simulink model "ACStesbed"  (R2015b)
settings: Solver=ode45  StartTime=0.0  StopTime=1500  FixedStep=0.02  RelTol=1e-3
StartFcn:
  | InitializeModel
values from neighbouring files (symbols this model uses):
  D = L+eye(3)    [controllability.m]    (also in func.m = skewsym(X(2:4))+eye(3); func1.m = skewsym(X(2:4))+eye(3); kab2.m = Dt'; sys1.m = skewsym(X0(2:4))+eye(3))
undefined symbols (not defined in the file or in its folder): DiscIntNeverNeededParam, e0_0, e1_0, e2_0, e3_0, OrbData, params
libraries: aerolibutil x16, vrlib x13, satellite_control_lib x8, dspmtrx3 x4, aerolibtransform2 x3, aerolib6dofsys x2, simulink x2, aerolib6dof2 x1, dspinverses x1, dspmathops x1
(part 1 of 2)
settings Model: Creator=DNikolaev  LastModifiedBy=DNikolaev
settings DataIOCC: SaveFormat=Array
settings DebuggingCC: UnderspecifiedInitializationDetection=Classic  MergeDetectMultiDrivingBlocksExec=none  SolverPrmCheckMsg=warning
settings HardwareCC: ProdBitPerPointer=32  ProdLargestAtomicFloat=None  ProdIntDivRoundTo=Undefined  ProdEndianess=Unspecified  ProdWordSize=32  ProdHWDeviceType=32-bit Generic
settings GRTTargetCC: GeneratePreprocessorConditionals=Disable all
settings ConfigComp: CovModelRefEnable=Off

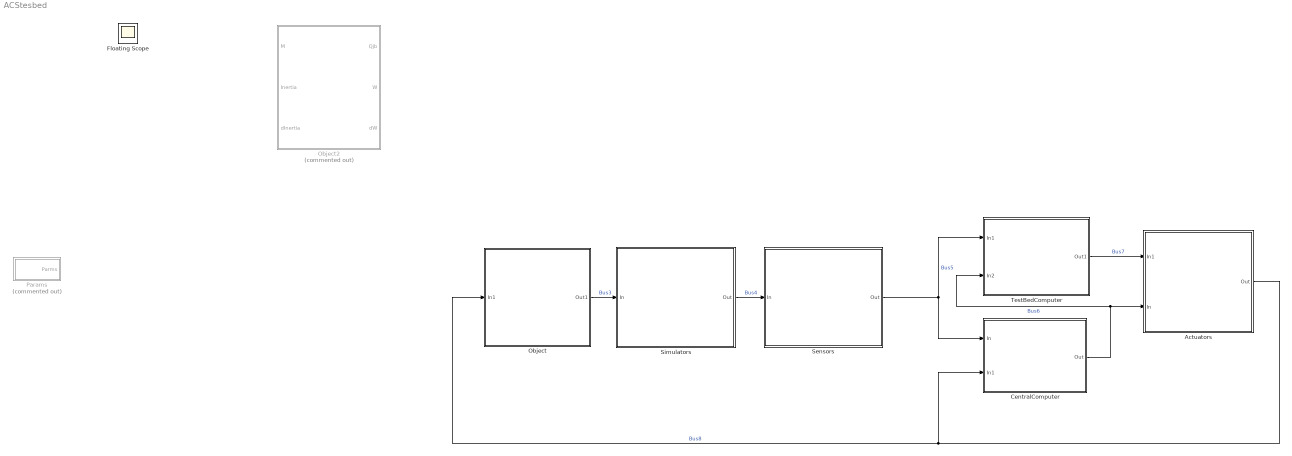
== system ACStesbed ==
  Actuators : Subsystem
      mask Display: image('ReactionWheel.gif','center','off')
  CentralComputer : Subsystem
      mask Display: image('cc.jpg')
  Object : Subsystem
      mask Display: image('abtestbed.jpg')
  Object2 : Subsystem  Commented=on
      mask Display: image('abtestbed.jpg')
  Params : Subsystem  Commented=on
  Sensors : Subsystem
      mask Display: image('gyro.jpg')
  Simulators : Subsystem
      mask Display: image('space.jpg')
  TestBedComputer : Subsystem  TreatAsAtomicUnit=on  SystemSampleTime=0.1
      mask Display: image('computer.jpg')
  Floating Scope : Scope
  wires:
  Simulators/1(Out) -> Sensors/1(In)  "Bus4"
  Sensors/1(Out) -> CentralComputer/1(In), TestBedComputer/1(In1)  "Bus5"
  Actuators/1(Out) -> Object/1(In1), CentralComputer/2(In1)  "Bus8"
  CentralComputer/1(Out) -> TestBedComputer/2(In2), Actuators/2(In)  "Bus6"
  TestBedComputer/1(Out1) -> Actuators/1(In1)  "Bus7"
  Object/1(Out1) -> Simulators/1(In)  "Bus3"

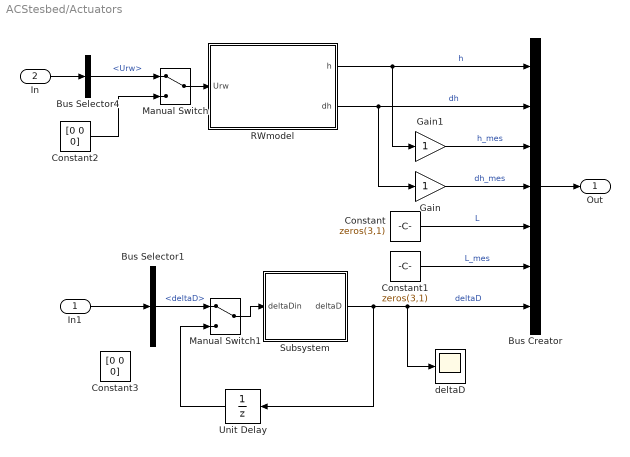
== system ACStesbed/Actuators ==
  In1 : Inport
  In : Inport  Port=2
  Bus Creator : BusCreator  Inputs=7
  Bus Selector1 : BusSelector  OutputSignals=deltaD
  Bus Selector4 : BusSelector  OutputSignals=Urw
  Constant : Constant  Value=zeros(3,1)
  Constant1 : Constant  Value=zeros(3,1)
  Constant2 : Constant  Value=[0 0 0]
  Constant3 : Constant  Value=[0 0 0]
  Gain : Gain
  Gain1 : Gain
  Manual Switch : ManualSwitch
  Manual Switch1 : ManualSwitch
  RWmodel : Subsystem
  Subsystem : Subsystem
  Unit Delay : UnitDelay  InitialCondition=[0 0 0]  SampleTime=-1
  deltaD : Scope
  Out : Outport
  wires:
  In/1 -> Bus Selector4/1
  Bus Creator/1 -> Out/1
  RWmodel/2(dh) -> Gain/1, Bus Creator/2  "dh"
  Constant/1 -> Bus Creator/5  "L"
  Constant1/1 -> Bus Creator/6  "L_mes"
  Subsystem/1(deltaD) -> Unit Delay/1, Bus Creator/7, deltaD/1  "deltaD"
  Bus Selector4/1 -> Manual Switch/1  "<Urw>"
  RWmodel/1(h) -> Bus Creator/1, Gain1/1  "h"
  Gain/1 -> Bus Creator/4  "dh_mes"
  Gain1/1 -> Bus Creator/3  "h_mes"
  In1/1 -> Bus Selector1/1
  Bus Selector1/1 -> Manual Switch1/1  "<deltaD>"
  Manual Switch/1 -> RWmodel/1(Urw)
  Constant2/1 -> Manual Switch/2
  Manual Switch1/1 -> Subsystem/1(deltaDin)
  Unit Delay/1 -> Manual Switch1/2

== system ACStesbed/CentralComputer ==
  In : Inport
  In1 : Inport  Port=2
  Bus Creator : BusCreator  Inputs=7
  Bus Selector : BusSelector  OutputSignals=W_mes,rj2000_mes,vj2000_mes,Qjb_starmes,B_mes,Sun_mag_angle_mes
  Bus Selector1 : BusSelector  OutputSignals=deltaD,h_mes,dh_mes
  ModelOfObject : Subsystem
  SPAttitude : Subsystem  Commented=on
  SatAttitude : Subsystem
  Out : Outport
  wires:
  In/1 -> Bus Selector/1
  Bus Creator/1 -> Out/1
  Bus Selector/1 -> SatAttitude/1(W_mes)  "<W_mes>"
  Bus Selector/2 -> SatAttitude/2(rj2000_mes)  "<rj2000_mes>"
  Bus Selector/3 -> SatAttitude/3(vj2000_mes)  "<vj2000_mes>"
  Bus Selector/4 -> SatAttitude/4(Qjb_starmes)  "<Qjb_starmes>"
  Bus Selector/5 -> SatAttitude/5(B_mes)  "<B_mes>"
  Bus Selector/6 -> SatAttitude/6(Rsun_mes)  "<Sun_mag_angle_mes>"
  ModelOfObject/1(J_est) -> Bus Creator/1, SatAttitude/7(J_mes)  "J_mes"
  SatAttitude/1(Urw) -> Bus Creator/2  "Urw"
  ModelOfObject/2(dJ_est) -> SatAttitude/8(dJ_mes)
  Bus Selector1/2 -> Bus Creator/7, SatAttitude/9(h_mes)  "<h_mes>"
  In1/1 -> Bus Selector1/1
  SatAttitude/3(Qjb_mes) -> Bus Creator/4  "Qjb_mes"
  SatAttitude/2(dW) -> Bus Creator/3  "dW"
  SatAttitude/4(Qob_mes) -> Bus Creator/5  "Qob_mes"
  Bus Selector1/1 -> ModelOfObject/1(deltaD)  "<deltaD>"
  Bus Selector1/3 -> Bus Creator/6  "<dh_mes>"

== system ACStesbed/Object ==
  In1 : Inport
  Bus Creator{,1..3} (4 alike) : BusCreator  Inputs=2
  Bus Selector : BusSelector  OutputSignals=Bus8.deltaD
  Bus Selector1 : BusSelector  OutputSignals=vj2000,j2000
  From Workspace : FromWorkspace  VariableName=InData  OutDataTypeStr=Bus: BusObject  SampleTime=0  OutputAfterFinalValue=Holding final value
  Inertia : Subsystem
  OrbitalBasis : Subsystem
  TestBedDynamics : Subsystem
      mask Display: image('abtestbed.jpg')
  Torques : Subsystem
  Out1 : Outport
  wires:
  TestBedDynamics/1(Qjb) -> Bus Creator/1  "Qjb"
  TestBedDynamics/2(Omega) -> Bus Creator/2  "W"
  Inertia/1(Inertia) -> TestBedDynamics/2(Inertia)
  Torques/1(T) -> TestBedDynamics/1(M)
  From Workspace/1 -> Bus Selector1/1, Bus Creator1/2  "Bus1"
  Bus Selector1/1 -> OrbitalBasis/1(vj2000)  "<vj2000>"
  Bus Selector1/2 -> OrbitalBasis/2(rj2000)  "<j2000>"
  Bus Creator/1 -> Bus Creator2/1, Bus Creator1/1
  Bus Creator1/1 -> Out1/1  "Bus3"
  Bus Creator2/1 -> Torques/1(InData)
  Inertia/2(dInertia) -> TestBedDynamics/3(dInertia)
  In1/1 -> Bus Creator3/1
  OrbitalBasis/1(Qjo) -> Bus Creator3/2
  Bus Creator3/1 -> Bus Selector/1, Bus Creator2/2
  Bus Selector/1 -> Inertia/1(deltaD)  "<deltaD>"

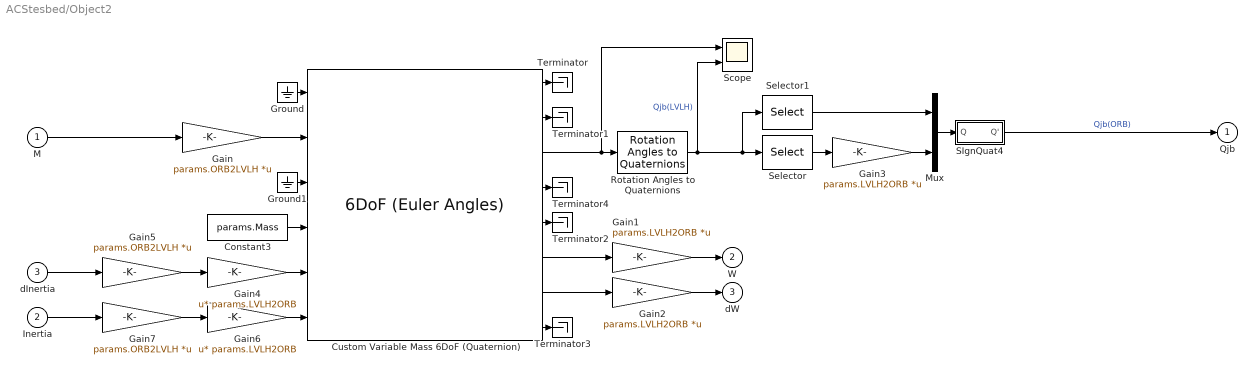
== system ACStesbed/Object2 ==
  M : Inport
  Inertia : Inport  Port=2
  dInertia : Inport  Port=3
  Constant3 : Constant  Value=params.Mass
  Custom Variable Mass 6DoF (Quaternion) : aerolib6dof2/6DoF (Euler Angles)  units=Metric (MKS)  mtype=Custom Variable  rep=Quaternion  xme_0=[0 0 0]  Vm_0=[0 0 0]  eul_0=[params.roll,params.pitch,params.yaw]  pm_0=params.ORB2LVLH*params.W_b  mass_0=1.0  mass_e=0  mass_f=0  inertia=eye(3)  inertia_e=eye(3)  inertia_f=eye(3)  k_quat=1.0
  Gain : Gain  Gain=params.ORB2LVLH  Multiplication=Matrix(K*u) (u vector)
  Gain1 : Gain  Gain=params.LVLH2ORB  Multiplication=Matrix(K*u) (u vector)
  Gain2 : Gain  Gain=params.LVLH2ORB  Multiplication=Matrix(K*u) (u vector)
  Gain3 : Gain  Gain=params.LVLH2ORB  Multiplication=Matrix(K*u) (u vector)
  Gain4 : Gain  Gain=params.LVLH2ORB  Multiplication=Matrix(u*K)
  Gain5 : Gain  Gain=params.ORB2LVLH  Multiplication=Matrix(K*u)
  Gain6 : Gain  Gain=params.LVLH2ORB  Multiplication=Matrix(u*K)
  Gain7 : Gain  Gain=params.ORB2LVLH  Multiplication=Matrix(K*u)
  Ground : Ground
  Ground1 : Ground
  Mux : Mux  Inputs=2
  Rotation Angles to Quaternions : aerolibtransform2/Rotation Angles to Quaternions  rotationOrder=XYZ
  SIgnQuat4 : Subsystem
  Scope : Scope  NumInputPorts=2
  Selector : Selector  InputPortWidth=4  IndexOptions=Index vector (dialog)  Indices=[2 3 4]  OutputSizes=1
  Selector1 : Selector  InputPortWidth=4  IndexOptions=Index vector (dialog)  Indices=1  OutputSizes=1
  Terminator{,1..4} (5 alike) : Terminator
  Qjb : Outport
  W : Outport  Port=2
  dW : Outport  Port=3
  wires:
  SIgnQuat4/1(Q') -> Qjb/1  "Qjb(ORB)"
  Mux/1 -> SIgnQuat4/1(Q)
  Constant3/1 -> Custom Variable Mass 6DoF (Quaternion)/4
  Gain6/1 -> Custom Variable Mass 6DoF (Quaternion)/6
  Gain7/1 -> Gain6/1
  Gain4/1 -> Custom Variable Mass 6DoF (Quaternion)/5
  Gain5/1 -> Gain4/1
  Gain3/1 -> Mux/2
  Selector1/1 -> Mux/1
  Selector/1 -> Gain3/1
  Inertia/1 -> Gain7/1
  Custom Variable Mass 6DoF (Quaternion)/3 -> Rotation Angles to Quaternions/1, Scope/1
  Gain2/1 -> dW/1
  Gain1/1 -> W/1
  Gain/1 -> Custom Variable Mass 6DoF (Quaternion)/2
  Custom Variable Mass 6DoF (Quaternion)/4 -> Terminator4/1
  dInertia/1 -> Gain5/1
  M/1 -> Gain/1
  Rotation Angles to Quaternions/1 -> Selector/1, Selector1/1, Scope/2  "Qjb(LVLH)"
  Custom Variable Mass 6DoF (Quaternion)/8 -> Terminator3/1
  Ground/1 -> Custom Variable Mass 6DoF (Quaternion)/1
  Custom Variable Mass 6DoF (Quaternion)/5 -> Terminator2/1
  Custom Variable Mass 6DoF (Quaternion)/1 -> Terminator/1
  Custom Variable Mass 6DoF (Quaternion)/7 -> Gain2/1
  Custom Variable Mass 6DoF (Quaternion)/6 -> Gain1/1
  Ground1/1 -> Custom Variable Mass 6DoF (Quaternion)/3
  Custom Variable Mass 6DoF (Quaternion)/2 -> Terminator1/1

== system ACStesbed/Params ==
  Bus Creator : BusCreator  Inputs=6
  Constant : Constant  Value=params.invJ_b
  Constant1 : Constant  Value=params.J_b
  Constant2 : Constant  Value=params.Nob
  Constant3 : Constant  Value=params.Mass
  Constant5 : Constant  Value=params.W_b
  Parms : Outport
  wires:
  Bus Creator/1 -> Parms/1
  Constant5/1 -> Bus Creator/5  "W_b_0"
  Constant2/1 -> Bus Creator/4  "Nob_0"
  Constant1/1 -> Bus Creator/2  "Inertia_0"
  Constant/1 -> Bus Creator/1  "invInertia_0"
  Constant3/1 -> Bus Creator/3  "Mass"

== system ACStesbed/Sensors ==
  In : Inport
  Bus Creator : BusCreator  Inputs=6
  Bus Selector4 : BusSelector  OutputSignals=j2000,vj2000,W,B,Qjb,Rsun
  MagnSensor : Subsystem
  PositionSensor : Subsystem
  RateSensor : Subsystem
      mask Display: text(0.5,0.5,'\omega=(I_3+S)\omega^{true}+\beta^{true}+\eta_\nu','hor','center','texmode','on')
  SIgnQuat : Subsystem
  StarSensor : Subsystem
  SunSensor : Subsystem
  Out : Outport
  wires:
  Bus Creator/1 -> Out/1
  In/1 -> Bus Selector4/1
  Bus Selector4/3 -> RateSensor/1(W)  "<W>"
  Bus Selector4/4 -> MagnSensor/1(Bms)  "<B>"
  Bus Selector4/1 -> SunSensor/2(rj2000), PositionSensor/1(rj2000)  "<j2000>"
  Bus Selector4/2 -> PositionSensor/2(vj2000)  "<vj2000>"
  Bus Selector4/5 -> SunSensor/1(Qjb), StarSensor/1(Qjb)  "<Qjb>"
  StarSensor/1(Qjb_mes) -> SIgnQuat/1(Q)
  MagnSensor/1(B_mes) -> Bus Creator/4  "B_mes"
  RateSensor/1(W_mes) -> Bus Creator/3  "W_mes"
  PositionSensor/2(vj2000_mes) -> Bus Creator/2  "vj2000_mes"
  PositionSensor/1(rj2000_mes) -> Bus Creator/1  "rj2000_mes"
  SIgnQuat/1(Q') -> Bus Creator/5  "Qjb_starmes"
  Bus Selector4/6 -> SunSensor/3(Rsun)  "<Rsun>"
  SunSensor/1(Sun_mag_angle_mes) -> Bus Creator/6

== system ACStesbed/Simulators ==
  In : Inport
  Bus Creator : BusCreator  Inputs=7
  Bus Selector1 : BusSelector  OutputSignals=signal1.W,signal1.Qjb
  Bus Selector4 : BusSelector  OutputSignals=Bus1.vj2000,Bus1.j2000,Bus1.rsun
  MagnSim : Subsystem
  StarSim : Subsystem
  SunSim : Subsystem
  Out : Outport
  wires:
  Bus Selector4/1 -> Bus Creator/1  "<vj2000>"
  In/1 -> Bus Selector1/1, Bus Selector4/1
  Bus Selector4/2 -> MagnSim/1(j2000), Bus Creator/2  "<j2000>"
  StarSim/1(Out) -> Bus Creator/3  "Stars"
  MagnSim/1(B) -> Bus Creator/4  "B"
  SunSim/1(Rsun_out) -> Bus Creator/5  "Rsun"
  Bus Creator/1 -> Out/1
  Bus Selector4/3 -> SunSim/1(Rsun)  "<rsun>"
  Bus Selector1/1 -> Bus Creator/6  "<W>"
  Bus Selector1/2 -> StarSim/1(In), Bus Creator/7  "<Qjb>"

== system ACStesbed/TestBedComputer ==
  In1 : Inport
  In2 : Inport  Port=2
  Bus Creator2 : BusCreator  Inputs=1
  Bus Selector3 : BusSelector  OutputSignals=rj2000_mes,vj2000_mes,W_mes
  Bus Selector4 : BusSelector  OutputSignals=Qob_mes,J_mes,dW,Urw,dh_mes,h_mes
  Constant8 : Constant  Value=params.g
  HorEst : Subsystem
  Mux : Mux  Inputs=2
  Quaternion Rotation2 : aerolibutil/Quaternion Rotation
  VerEst : Subsystem
  Out1 : Outport
  wires:
  In1/1 -> Bus Selector3/1
  In2/1 -> Bus Selector4/1
  Bus Creator2/1 -> Out1/1
  Mux/1 -> Bus Creator2/1  "deltaD"
  Bus Selector4/1 -> Quaternion Rotation2/1  "<Qob_mes>"
  Bus Selector4/3 -> HorEst/2(dW)  "<dW>"
  HorEst/1(deltaD12) -> Mux/1
  Constant8/1 -> Quaternion Rotation2/2  "g"
  Quaternion Rotation2/1 -> VerEst/1(gb), HorEst/1(gb)
  Bus Selector4/4 -> ?  "<Urw>"
  Bus Selector4/2 -> VerEst/2(J)  "<J_mes>"
  Bus Selector4/5 -> VerEst/3(dh)  "<dh_mes>"
  Bus Selector4/6 -> VerEst/4(h)  "<h_mes>"
  Bus Selector3/3 -> VerEst/5(W)  "<W_mes>"
  VerEst/1(Rz_est) -> ?  "Rz_est"

== system ACStesbed/Actuators/RWmodel ==
  Urw : Inport
  Gain1 : Gain
  Integrator Limited : Integrator  InitialCondition=[0 0 0]  LimitOutput=on  UpperSaturationLimit=100  LowerSaturationLimit=-100
  Rate Transition : RateTransition  OutPortSampleTime=0.01
  Saturation : Saturate
  "dh, h" : Scope  NumInputPorts=2
  h : Outport
  dh : Outport  Port=2
  wires:
  Urw/1 -> Rate Transition/1
  Integrator Limited/1 -> "dh, h"/2, h/1  "h"
  Gain1/1 -> Saturation/1  "dh"
  Saturation/1 -> dh/1
  Rate Transition/1 -> "dh, h"/1, Gain1/1, Integrator Limited/1  "dh"

== system ACStesbed/Actuators/Subsystem ==
  deltaDin : Inport
  Rate Transition : RateTransition  OutPortSampleTime=0.01
  deltaD : Outport
  wires:
  Rate Transition/1 -> deltaD/1  "deltaD"
  deltaDin/1 -> Rate Transition/1

== system ACStesbed/CentralComputer/ModelOfObject ==
  deltaD : Inport
  ChangeMe1 : Constant  Value=zeros(3,3)
  ChangeMe4 : Constant  Value=zeros(3,3)
  Inertia : Subsystem
  J_est : Outport
  dJ_est : Outport  Port=2
  R_est : Outport  Port=3
  wires:
  deltaD/1 -> Inertia/1(deltaD)
  ChangeMe1/1 -> dJ_est/1
  Inertia/1(Inertia) -> J_est/1
  ChangeMe4/1 -> R_est/1

== system ACStesbed/CentralComputer/SPAttitude ==
  In1 : Inport
  Out1 : Outport
  wires:
  In1/1 -> Out1/1

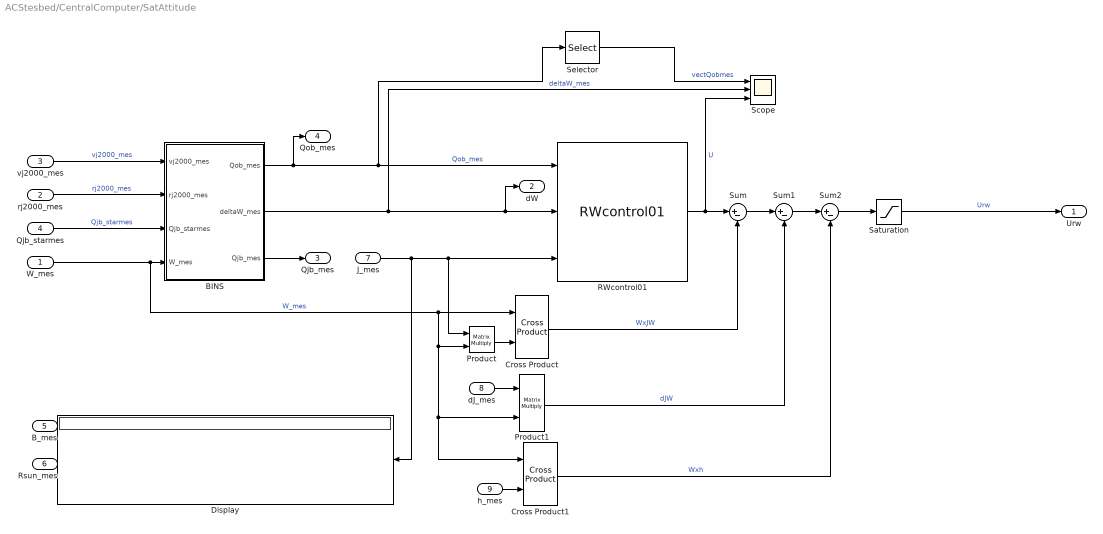
== system ACStesbed/CentralComputer/SatAttitude ==
  W_mes : Inport
  rj2000_mes : Inport  Port=2
  vj2000_mes : Inport  Port=3
  Qjb_starmes : Inport  Port=4
  B_mes : Inport  Port=5
  Rsun_mes : Inport  Port=6
  J_mes : Inport  Port=7
  dJ_mes : Inport  Port=8
  h_mes : Inport  Port=9
  BINS : Subsystem
  Cross Product : vrlib/Utilities/Cross Product
  Cross Product1 : vrlib/Utilities/Cross Product
  Display : Display
  Product : Product  Multiplication=Matrix(*)
  Product1 : Product  Multiplication=Matrix(*)
  RWcontrol01 : satellite_control_lib/RWcontrol01  Kq=params.K1acs  Kw=params.K2acs
  Saturation : Saturate
  Scope : Scope  NumInputPorts=3
  Selector : Selector  InputPortWidth=4  IndexOptions=Index vector (dialog)  Indices=[2 3 4]  OutputSizes=1
  Sum : Sum  Inputs=|+-
  Sum1 : Sum  Inputs=|+-
  Sum2 : Sum  Inputs=|+-
  Urw : Outport
  dW : Outport  Port=2
  Qjb_mes : Outport  Port=3
  Qob_mes : Outport  Port=4
  wires:
  RWcontrol01/1 -> Scope/3, Sum/1  "U"
  vj2000_mes/1 -> BINS/1(vj2000_mes)  "vj2000_mes"
  rj2000_mes/1 -> BINS/2(rj2000_mes)  "rj2000_mes"
  Qjb_starmes/1 -> BINS/3(Qjb_starmes)  "Qjb_starmes"
  W_mes/1 -> Product/2, Product1/2, Cross Product1/1, Cross Product/1, BINS/4(W_mes)  "W_mes"
  J_mes/1 -> Display/1, Product/1, RWcontrol01/3
  BINS/1(Qob_mes) -> Qob_mes/1, Selector/1, RWcontrol01/1  "Qob_mes"
  BINS/2(deltaW_mes) -> Scope/2, dW/1, RWcontrol01/2  "deltaW_mes"
  Product/1 -> Cross Product/2
  Cross Product/1 -> Sum/2  "WxJW"
  Product1/1 -> Sum1/2  "dJW"
  Cross Product1/1 -> Sum2/2  "Wxh"
  Sum/1 -> Sum1/1
  Sum1/1 -> Sum2/1
  Sum2/1 -> Saturation/1
  h_mes/1 -> Cross Product1/2
  dJ_mes/1 -> Product1/1
  BINS/3(Qjb_mes) -> Qjb_mes/1
  Saturation/1 -> Urw/1  "Urw"
  Selector/1 -> Scope/1  "vectQobmes"

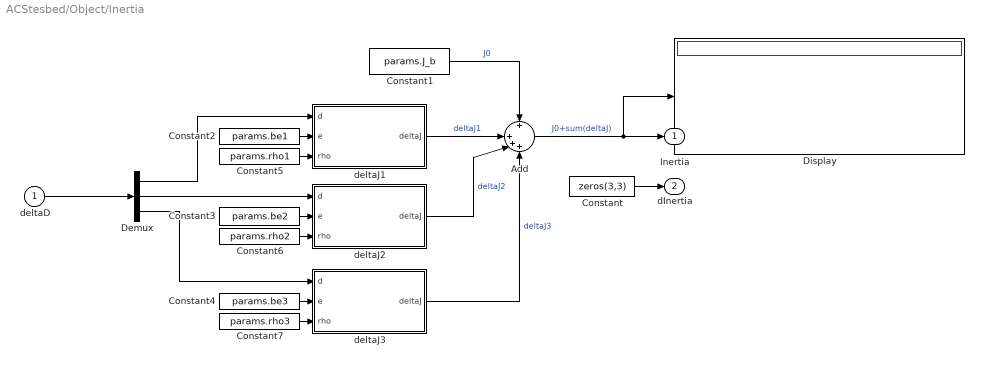
== system ACStesbed/Object/Inertia ==
  deltaD : Inport
  Add : Sum  Inputs=+|+++
  Constant : Constant  Value=zeros(3,3)
  Constant1 : Constant  Value=params.J_b
  Constant2 : Constant  Value=params.be1
  Constant3 : Constant  Value=params.be2
  Constant4 : Constant  Value=params.be3
  Constant5 : Constant  Value=params.rho1
  Constant6 : Constant  Value=params.rho2
  Constant7 : Constant  Value=params.rho3
  Demux : Demux  Outputs=3
  Display : Display
  deltaJ1 : Subsystem
  deltaJ2 : Subsystem
  deltaJ3 : Subsystem
  Inertia : Outport
  dInertia : Outport  Port=2
  wires:
  Constant/1 -> dInertia/1
  Constant1/1 -> Add/1  "J0"
  deltaD/1 -> Demux/1
  deltaJ1/1(deltaJ) -> Add/2  "deltaJ1"
  deltaJ2/1(deltaJ) -> Add/3  "deltaJ2"
  deltaJ3/1(deltaJ) -> Add/4  "deltaJ3"
  Add/1 -> Display/1, Inertia/1  "J0+sum(deltaJ)"
  Demux/1 -> deltaJ1/1(d)
  Demux/2 -> deltaJ2/1(d)
  Demux/3 -> deltaJ3/1(d)
  Constant4/1 -> deltaJ3/2(e)
  Constant3/1 -> deltaJ2/2(e)
  Constant2/1 -> deltaJ1/2(e)
  Constant7/1 -> deltaJ3/3(rho)
  Constant6/1 -> deltaJ2/3(rho)
  Constant5/1 -> deltaJ1/3(rho)

== system ACStesbed/Object/OrbitalBasis ==
  vj2000 : Inport
  rj2000 : Inport  Port=2
  Cross Product : vrlib/Utilities/Cross Product
  Cross Product1 : vrlib/Utilities/Cross Product
  Direction Cosine Matrix to Quaternions : aerolibtransform2/Direction Cosine Matrix  to Quaternions
  Matrix Concatenate : Concatenate  NumInputs=3  Mode=Multidimensional array  ConcatenateDimension=2
  Normalize Vector : vrlib/Utilities/Normalize Vector  maxzero=0.00001
  Normalize Vector1 : vrlib/Utilities/Normalize Vector  maxzero=0.00001
  Quaternion Conjugate : aerolibutil/Quaternion Conjugate
  Qjo : Outport
  wires:
  Cross Product1/1 -> Matrix Concatenate/1  "iorb"
  Normalize Vector/1 -> Matrix Concatenate/2, Cross Product1/1  "jorb"
  Matrix Concatenate/1 -> Direction Cosine Matrix to Quaternions/1  "DCMjo"
  rj2000/1 -> Normalize Vector/1, Cross Product/2
  vj2000/1 -> Cross Product/1
  Direction Cosine Matrix to Quaternions/1 -> Quaternion Conjugate/1  "Qjo(in J frame)"
  Normalize Vector1/1 -> Matrix Concatenate/3, Cross Product1/2  "korb"
  Cross Product/1 -> Normalize Vector1/1
  Quaternion Conjugate/1 -> Qjo/1  "Qjo"

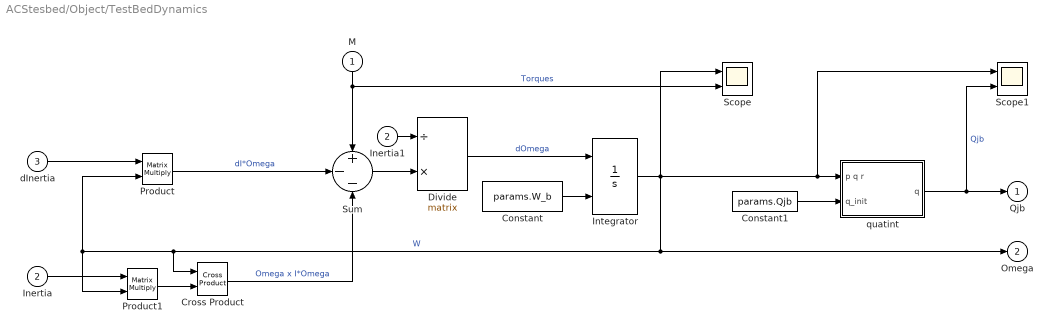
== system ACStesbed/Object/TestBedDynamics ==
  M : Inport
  Inertia : Inport  Port=2
  dInertia : Inport  Port=3
  Constant : Constant  Value=params.W_b
  Constant1 : Constant  Value=params.Qjb
  Cross Product : vrlib/Utilities/Cross Product
  Divide : Product  Inputs=/*  Multiplication=Matrix(*)
  Inertia1 : InportShadow  Port=2
  Integrator : Integrator  InitialConditionSource=external
  Product : Product  Multiplication=Matrix(*)
  Product1 : Product  Multiplication=Matrix(*)
  Scope : Scope  NumInputPorts=2
  Scope1 : Scope  NumInputPorts=2
  Sum : Sum  Inputs=+--
  quatint : Subsystem
  Qjb : Outport
  Omega : Outport  Port=2
  wires:
  Sum/1 -> Divide/2
  Inertia1/1 -> Divide/1
  Divide/1 -> Integrator/1  "dOmega"
  Constant/1 -> Integrator/2
  Product/1 -> Sum/2  "dI*Omega"
  dInertia/1 -> Product/1
  Constant1/1 -> quatint/2(q_init)
  quatint/1(q) -> Scope1/2, Qjb/1  "Qjb"
  Inertia/1 -> Product1/1
  Product1/1 -> Cross Product/2
  Cross Product/1 -> Sum/3  "Omega x I*Omega"
  Integrator/1 -> Scope/1, Scope1/1, quatint/1(p q r), Cross Product/1, Product/2, Product1/2, Omega/1  "W"
  M/1 -> Scope/2, Sum/1  "Torques"

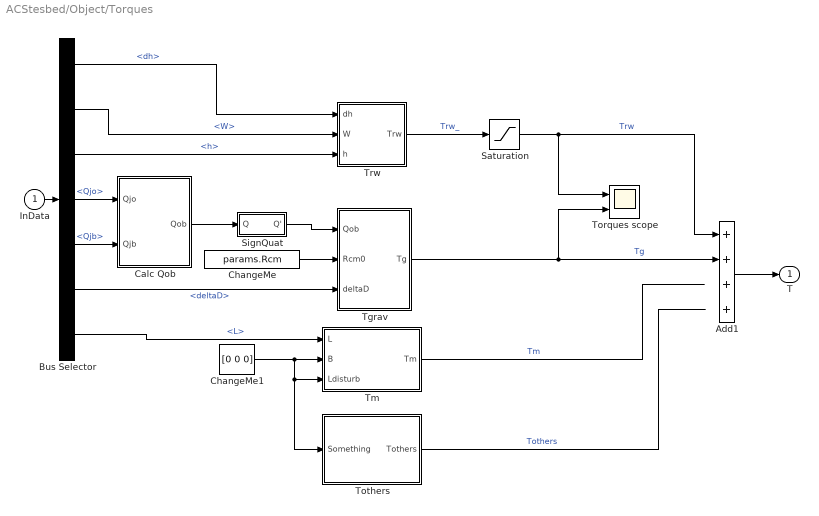
== system ACStesbed/Object/Torques ==
  InData : Inport
  Add1 : Sum  Inputs=4
  Bus Selector : BusSelector  OutputSignals=signal2.Bus8.dh,signal1.W,signal2.Bus8.h,signal2.Qjo,signal1.Qjb,signal2.Bus8.deltaD,signal2.Bus8.L
  Calc Qob : Subsystem
  ChangeMe : Constant  Value=params.Rcm
  ChangeMe1 : Constant  Value=[0 0 0]
  Saturation : Saturate  UpperLimit=1  LowerLimit=-1
  SignQuat : Subsystem
  Tgrav : Subsystem
  Tm : Subsystem
  Torques scope : Scope  NumInputPorts=2
  Tothers : Subsystem
  Trw : Subsystem
  T : Outport
  wires:
  InData/1 -> Bus Selector/1
  Bus Selector/7 -> Tm/1(L)  "<L>"
  Bus Selector/6 -> Tgrav/3(deltaD)  "<deltaD>"
  Add1/1 -> T/1
  Bus Selector/1 -> Trw/1(dh)  "<dh>"
  Bus Selector/2 -> Trw/2(W)  "<W>"
  Bus Selector/3 -> Trw/3(h)  "<h>"
  Trw/1(Trw) -> Saturation/1  "Trw_"
  Tgrav/1(Tg) -> Torques scope/2, Add1/2  "Tg"
  Tm/1(Tm) -> ?  "Tm"
  Tothers/1(Tothers) -> ?  "Tothers"
  ChangeMe1/1 -> Tothers/1(Something), Tm/3(Ldisturb), Tm/2(B)
  Saturation/1 -> Torques scope/1, Add1/1  "Trw"
  ChangeMe/1 -> Tgrav/2(Rcm0)
  Calc Qob/1(Qob) -> SignQuat/1(Q)
  Bus Selector/5 -> Calc Qob/2(Qjb)  "<Qjb>"
  Bus Selector/4 -> Calc Qob/1(Qjo)  "<Qjo>"
  SignQuat/1(Q') -> Tgrav/1(Qob)

== system ACStesbed/Object2/SIgnQuat4 ==
  Q : Inport
  Constant : Constant
  Constant1 : Constant  Value=-1
  Product : Product
  Selector2 : Selector  InputPortWidth=4  IndexOptions=Index vector (dialog)  Indices=[1]  OutputSizes=1
  Switch : Switch
  Q' : Outport
  wires:
  Constant1/1 -> Switch/3
  Constant/1 -> Switch/1
  Selector2/1 -> Switch/2
  Switch/1 -> Product/1
  Product/1 -> Q'/1
  Q/1 -> Selector2/1, Product/2

== system ACStesbed/Sensors/MagnSensor ==
  note: B_mes=A*B+b+w
  Bms : Inport
  A : Constant  Value=diag([1 1 1])
  Matrix Multiply : Product  Multiplication=Matrix(*)
  Random Noise : RandomNumber  Variance=params.MS_varianse  SampleTime=params.MS_sample_time
  Reshape : Reshape  OutputDimensionality=Column vector (2-D)
  Sum : Sum  Inputs=|++
  Sum1 : Sum  Inputs=|++
  Zero-Order Hold : ZeroOrderHold  SampleTime=params.SS_sample_time
  b : Constant  Value=[0;0;0]
  B_mes : Outport
  wires:
  Random Noise/1 -> Sum/2  "w"
  Bms/1 -> Zero-Order Hold/1
  Sum/1 -> B_mes/1  "B_mes"
  A/1 -> Matrix Multiply/1  "A"
  Matrix Multiply/1 -> Sum1/1
  Reshape/1 -> Matrix Multiply/2  "B"
  b/1 -> Sum1/2  "b"
  Zero-Order Hold/1 -> Reshape/1
  Sum1/1 -> Sum/1

== system ACStesbed/Sensors/PositionSensor ==
  rj2000 : Inport
  vj2000 : Inport  Port=2
  Noise : Constant  Value=[0 0 0]
  Noise1 : Constant  Value=[0 0 0]
  Sum : Sum  Inputs=|++
  Sum1 : Sum  Inputs=|++
  Zero-Order Hold : ZeroOrderHold  SampleTime=0.1
  Zero-Order Hold1 : ZeroOrderHold  SampleTime=0.1
  rj2000_mes : Outport
  vj2000_mes : Outport  Port=2
  wires:
  rj2000/1 -> Sum/1
  Noise/1 -> Sum/2
  Sum/1 -> Zero-Order Hold/1
  Zero-Order Hold/1 -> rj2000_mes/1
  vj2000/1 -> Sum1/1
  Noise1/1 -> Sum1/2
  Sum1/1 -> Zero-Order Hold1/1
  Zero-Order Hold1/1 -> vj2000_mes/1

== system ACStesbed/Sensors/RateSensor ==
  W : Inport
  Add : Sum
  Band-Limited White Noise : simulink/Sources/Band-Limited White Noise  Cov=params.VarRSB/0.1  Ts=0.1  seed=[23341]
  Band-Limited White Noise1 : simulink/Sources/Band-Limited White Noise  Cov=params.VarRSN/0.1  Ts=0.1  seed=[23341]
  Constant : Constant  Value=params.RSSE
  I3 : dspmtrx3/Constant Diagonal Matrix  q=ones(1,3)  frame=off  dataType=Inherit from 'Constant(s) along diagonal'  isSigned=on  wordLen=16  udDataType=sfix(16)  fracBitsMode=Best precision  numFracBits=15
  Integrator : Integrator
  Manual Switch : ManualSwitch
  Product : Product  Multiplication=Matrix(*)
  Sum : Sum  Inputs=|++
  Sum1 : Sum  Inputs=|++
  Zero-Order Hold : ZeroOrderHold  SampleTime=0.1
  Zero-Order Hold1 : ZeroOrderHold  SampleTime=0.1
  W_mes : Outport
  wires:
  W/1 -> Zero-Order Hold1/1, Product/2
  Sum/1 -> Zero-Order Hold/1
  Zero-Order Hold/1 -> Manual Switch/2
  Sum1/1 -> Sum/1
  I3/1 -> Add/1
  Constant/1 -> Add/2
  Add/1 -> Product/1
  Product/1 -> Sum1/1
  Band-Limited White Noise1/1 -> Sum/2  "noise"
  Integrator/1 -> Sum1/2  "Bias"
  Band-Limited White Noise/1 -> Integrator/1  "dBias"
  Manual Switch/1 -> W_mes/1
  Zero-Order Hold1/1 -> Manual Switch/1

== system ACStesbed/Sensors/SIgnQuat ==
  Q : Inport
  Product : Product
  Selector2 : Selector  InputPortWidth=4  IndexOptions=Index vector (dialog)  Indices=[1]  OutputSizes=1
  Sign : Signum
  Q' : Outport
  wires:
  Q/1 -> Product/2, Selector2/1
  Product/1 -> Q'/1
  Sign/1 -> Product/1
  Selector2/1 -> Sign/1

== system ACStesbed/Sensors/StarSensor ==
  Qjb : Inport
  Noise : Constant  Value=[1 0 0 0]
  Quaternion Multiplication : aerolibutil/Quaternion Multiplication
  Zero-Order Hold : ZeroOrderHold  SampleTime=0.1
  Qjb_mes : Outport
  wires:
  Zero-Order Hold/1 -> Qjb_mes/1
  Qjb/1 -> Quaternion Multiplication/1
  Noise/1 -> Quaternion Multiplication/2
  Quaternion Multiplication/1 -> Zero-Order Hold/1

== system ACStesbed/Sensors/SunSensor ==
  Qjb : Inport
  rj2000 : Inport  Port=2
  Rsun : Inport  Port=3
  Constant : Constant  Value=params.Qb_ss
  DigitalSunSensor : Subsystem
  Gain : Gain  Gain=params.au2km
  Quaternion Multiplication : aerolibutil/Quaternion Multiplication
  Quaternion Rotation : aerolibutil/Quaternion Rotation
  Subtract : Sum  Inputs=|+-
  Sun_mag_angle_mes : Outport
  wires:
  Quaternion Rotation/1 -> DigitalSunSensor/1(Rsun_ss)  "Rsun_ss"
  Gain/1 -> Subtract/1
  Subtract/1 -> Quaternion Rotation/2  "Rsun_j"
  Quaternion Multiplication/1 -> Quaternion Rotation/1  "Qj_ss"
  Rsun/1 -> Gain/1
  DigitalSunSensor/1(Sun_mag_angle_mes) -> Sun_mag_angle_mes/1  "Sun_mag_angle_mes"
  Constant/1 -> Quaternion Multiplication/2
  rj2000/1 -> Subtract/2
  Qjb/1 -> Quaternion Multiplication/1

== system ACStesbed/Simulators/MagnSim ==
  j2000 : Inport
  B : Outport
  wires:
  j2000/1 -> B/1

== system ACStesbed/Simulators/StarSim ==
  In : Inport
  Out : Outport
  wires:
  In/1 -> Out/1

== system ACStesbed/Simulators/SunSim ==
  Rsun : Inport
  Rsun_out : Outport
  wires:
  Rsun/1 -> Rsun_out/1

== system ACStesbed/TestBedComputer/HorEst ==
  gb : Inport
  dW : Inport  Port=2
  Constant13 : Constant  Value=params.invU
  Gain : Gain  Gain=-params.Mass
  Gain1 : Gain  Gain=params.Mass/params.bmass+3
  Product8 : Product  Inputs=3  Multiplication=Matrix(*)
  Pseudoinverse : dspinverses/Pseudoinverse  wanterr=off
  Selector : Selector  InputPortWidth=3  IndexOptions=Index vector (dialog)  Indices=[1 2]  OutputSizes=1
  Skew-symmetric matrix2 : satellite_control_lib/Skew-symmetric matrix
  Subsystem : Subsystem
  deltaD HorEst : Scope
  tau_b : Scope
  deltaD12 : Outport
  wires:
  gb/1 -> Skew-symmetric matrix2/1, Subsystem/2(gb)  "gb"
  Skew-symmetric matrix2/1 -> Gain/1  "G"
  Pseudoinverse/1 -> Product8/2  "psinvG"
  dW/1 -> Subsystem/3(dW)
  Subsystem/1(taub) -> Product8/3, tau_b/1
  Constant13/1 -> Product8/1
  Product8/1 -> Gain1/1
  Selector/1 -> deltaD12/1
  Gain/1 -> Subsystem/1(G), Pseudoinverse/1  "G"
  Gain1/1 -> deltaD HorEst/1, Selector/1

== system ACStesbed/TestBedComputer/VerEst ==
  gb : Inport
  J : Inport  Port=2
  dh : Inport  Port=3
  h : Inport  Port=4
  W : Inport  Port=5
  Constant1 : Constant  Value=params.Mass
  Display : Display
  Scope : Scope
  Scope1 : Scope
  Unit Delay : UnitDelay  InitialCondition=0.001  SampleTime=-1
  Unit Delay1 : UnitDelay  InitialCondition=diag([1e-10,1e-10,1e-10,1e-50])  SampleTime=-1
  Unit Delay2 : UnitDelay  InitialCondition=[0 0 0]  SampleTime=-1
  Unscented Kalman Filter : MATLAB Function  TreatAsAtomicUnit=on
  Rz_est : Outport
  wires:
  gb/1 -> Unscented Kalman Filter/7(gb)
  Unit Delay2/1 -> Unscented Kalman Filter/3(W_estin)
  Constant1/1 -> Unscented Kalman Filter/9(Mass)
  dh/1 -> Unscented Kalman Filter/5(dh)
  J/1 -> Unscented Kalman Filter/8(J)
  Unscented Kalman Filter/1(rz_est) -> Unit Delay/1, Scope/1  "z_est"
  W/1 -> Unscented Kalman Filter/1(W)
  Unit Delay1/1 -> Unscented Kalman Filter/4(Pin)
  Unscented Kalman Filter/2(W_est) -> Unit Delay2/1, Scope1/1
  h/1 -> Unscented Kalman Filter/6(h)
  Unit Delay/1 -> Rz_est/1, Unscented Kalman Filter/2(rz_estin)
  Unscented Kalman Filter/3(P) -> Display/1, Unit Delay1/1

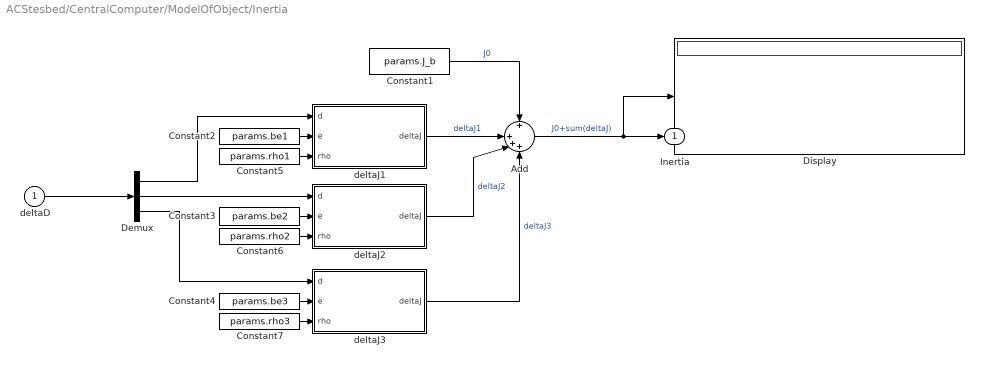
== system ACStesbed/CentralComputer/ModelOfObject/Inertia ==
  deltaD : Inport
  Add : Sum  Inputs=+|+++
  Constant1 : Constant  Value=params.J_b
  Constant2 : Constant  Value=params.be1
  Constant3 : Constant  Value=params.be2
  Constant4 : Constant  Value=params.be3
  Constant5 : Constant  Value=params.rho1
  Constant6 : Constant  Value=params.rho2
  Constant7 : Constant  Value=params.rho3
  Demux : Demux  Outputs=3
  Display : Display
  deltaJ1 : Subsystem
  deltaJ2 : Subsystem
  deltaJ3 : Subsystem
  Inertia : Outport
  wires:
  Constant1/1 -> Add/1  "J0"
  deltaD/1 -> Demux/1
  deltaJ1/1(deltaJ) -> Add/2  "deltaJ1"
  deltaJ2/1(deltaJ) -> Add/3  "deltaJ2"
  deltaJ3/1(deltaJ) -> Add/4  "deltaJ3"
  Add/1 -> Display/1, Inertia/1  "J0+sum(deltaJ)"
  Demux/1 -> deltaJ1/1(d)
  Demux/2 -> deltaJ2/1(d)
  Demux/3 -> deltaJ3/1(d)
  Constant4/1 -> deltaJ3/2(e)
  Constant3/1 -> deltaJ2/2(e)
  Constant2/1 -> deltaJ1/2(e)
  Constant7/1 -> deltaJ3/3(rho)
  Constant6/1 -> deltaJ2/3(rho)
  Constant5/1 -> deltaJ1/3(rho)

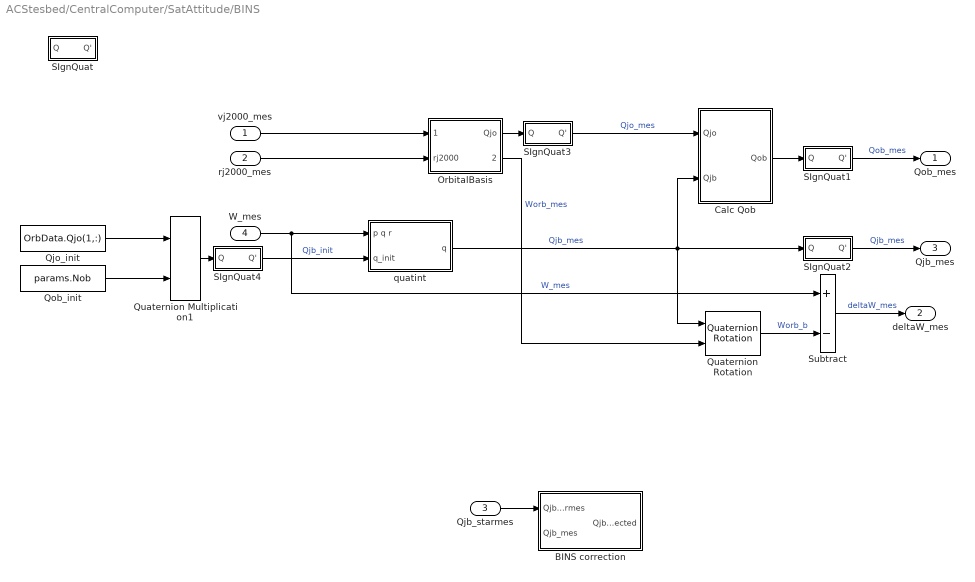
== system ACStesbed/CentralComputer/SatAttitude/BINS ==
  vj2000_mes : Inport
  rj2000_mes : Inport  Port=2
  Qjb_starmes : Inport  Port=3
  W_mes : Inport  Port=4
  BINS correction : Subsystem
  Calc Qob : Subsystem
  OrbitalBasis : Subsystem
  Qjo_init : Constant  Value=OrbData.Qjo(1,:)
  Qob_init : Constant  Value=params.Nob
  Quaternion Multiplication1 : aerolibutil/Quaternion Multiplication
  Quaternion Rotation : aerolibutil/Quaternion Rotation
  SIgnQuat : Subsystem
  SIgnQuat1 : Subsystem
  SIgnQuat2 : Subsystem
  SIgnQuat3 : Subsystem
  SIgnQuat4 : Subsystem
  Subtract : Sum  Inputs=+-
  quatint : Subsystem
  Qob_mes : Outport
  deltaW_mes : Outport  Port=2
  Qjb_mes : Outport  Port=3
  wires:
  Qjb_starmes/1 -> BINS correction/1(Qjb_starmes)
  quatint/1(q) -> SIgnQuat2/1(Q), Calc Qob/2(Qjb), Quaternion Rotation/1  "Qjb_mes"
  Calc Qob/1(Qob) -> SIgnQuat1/1(Q)
  rj2000_mes/1 -> OrbitalBasis/2(rj2000)
  vj2000_mes/1 -> OrbitalBasis/1(vj2000)
  OrbitalBasis/1(Qjo) -> SIgnQuat3/1(Q)
  OrbitalBasis/2(Worb_j) -> Quaternion Rotation/2  "Worb_mes"
  W_mes/1 -> Subtract/1, quatint/1(p q r)  "W_mes"
  Subtract/1 -> deltaW_mes/1  "deltaW_mes"
  Qjo_init/1 -> Quaternion Multiplication1/1
  Qob_init/1 -> Quaternion Multiplication1/2
  Quaternion Multiplication1/1 -> SIgnQuat4/1(Q)
  Quaternion Rotation/1 -> Subtract/2  "Worb_b"
  SIgnQuat1/1(Q') -> Qob_mes/1  "Qob_mes"
  SIgnQuat2/1(Q') -> Qjb_mes/1  "Qjb_mes"
  SIgnQuat3/1(Q') -> Calc Qob/1(Qjo)  "Qjo_mes"
  SIgnQuat4/1(Q') -> quatint/2(q_init)  "Qjb_init"

== system ACStesbed/Object/Inertia/deltaJ1 ==
  d : Inport
  e : Inport  Port=2
  rho : Inport  Port=3
  Add : Sum
  Constant : Constant  Value=params.bmass
  Gain : Gain  Gain=-1
  Product : Product  Inputs=3
  Product1 : Product
  Skew-symmetric matrix : satellite_control_lib/Skew-symmetric matrix
  deltaJ : Outport
  wires:
  Constant/1 -> Gain/1
  e/1 -> Product1/2
  rho/1 -> Add/2
  Product/1 -> deltaJ/1  "(-m)[R x][R x]"
  Gain/1 -> Product/1
  d/1 -> Product1/1
  Product1/1 -> Add/1
  Add/1 -> Skew-symmetric matrix/1  "R"
  Skew-symmetric matrix/1 -> Product/3, Product/2

== system ACStesbed/Object/Inertia/deltaJ2 ==
  d : Inport
  e : Inport  Port=2
  rho : Inport  Port=3
  Add : Sum
  Constant : Constant  Value=params.bmass
  Gain : Gain  Gain=-1
  Product : Product  Inputs=3
  Product1 : Product
  Skew-symmetric matrix : satellite_control_lib/Skew-symmetric matrix
  deltaJ : Outport
  wires:
  Skew-symmetric matrix/1 -> Product/2, Product/3
  Add/1 -> Skew-symmetric matrix/1  "R"
  Product1/1 -> Add/1
  d/1 -> Product1/1
  Gain/1 -> Product/1
  Product/1 -> deltaJ/1  "(-m)[R x][R x]"
  rho/1 -> Add/2
  e/1 -> Product1/2
  Constant/1 -> Gain/1

== system ACStesbed/Object/Inertia/deltaJ3 ==
  d : Inport
  e : Inport  Port=2
  rho : Inport  Port=3
  Add : Sum
  Constant : Constant  Value=params.bmass
  Gain : Gain  Gain=-1
  Product : Product  Inputs=3
  Product1 : Product
  Skew-symmetric matrix : satellite_control_lib/Skew-symmetric matrix
  deltaJ : Outport
  wires:
  Constant/1 -> Gain/1
  e/1 -> Product1/2
  rho/1 -> Add/2
  Product/1 -> deltaJ/1  "(-m)[R x][R x]"
  Gain/1 -> Product/1
  d/1 -> Product1/1
  Product1/1 -> Add/1
  Add/1 -> Skew-symmetric matrix/1  "R"
  Skew-symmetric matrix/1 -> Product/3, Product/2

== system ACStesbed/Object/TestBedDynamics/quatint ==
  p q r : Inport
  q_init : Inport  Port=2
  q0 q1 q2 q3 : Integrator  InitialConditionSource=external  InitialCondition=[e0_0 e1_0 e2_0 e3_0]
  qdot : aerolib6dofsys/DCM & Euler Angles (Quaternion)/qdot
  q : Outport
  wires:
  q0 q1 q2 q3/1 -> q/1, qdot/2
  q_init/1 -> q0 q1 q2 q3/2
  p q r/1 -> qdot/1
  qdot/1 -> q0 q1 q2 q3/1

== system ACStesbed/Object/Torques/Calc Qob ==
  Qjo : Inport
  Qjb : Inport  Port=2
  Quaternion Inverse : aerolibutil/Quaternion Inverse
  Quaternion Multiplication : aerolibutil/Quaternion Multiplication
  Qob : Outport
  wires:
  Qjb/1 -> Quaternion Multiplication/2  "Qjb"
  Qjo/1 -> Quaternion Inverse/1  "Qjo"
  Quaternion Inverse/1 -> Quaternion Multiplication/1
  Quaternion Multiplication/1 -> Qob/1

== system ACStesbed/Object/Torques/SignQuat ==
  Q : Inport
  Product : Product
  Selector2 : Selector  InputPortWidth=4  IndexOptions=Index vector (dialog)  Indices=[1]  OutputSizes=1
  Sign : Signum
  Q' : Outport
  wires:
  Q/1 -> Product/2, Selector2/1
  Product/1 -> Q'/1
  Sign/1 -> Product/1
  Selector2/1 -> Sign/1

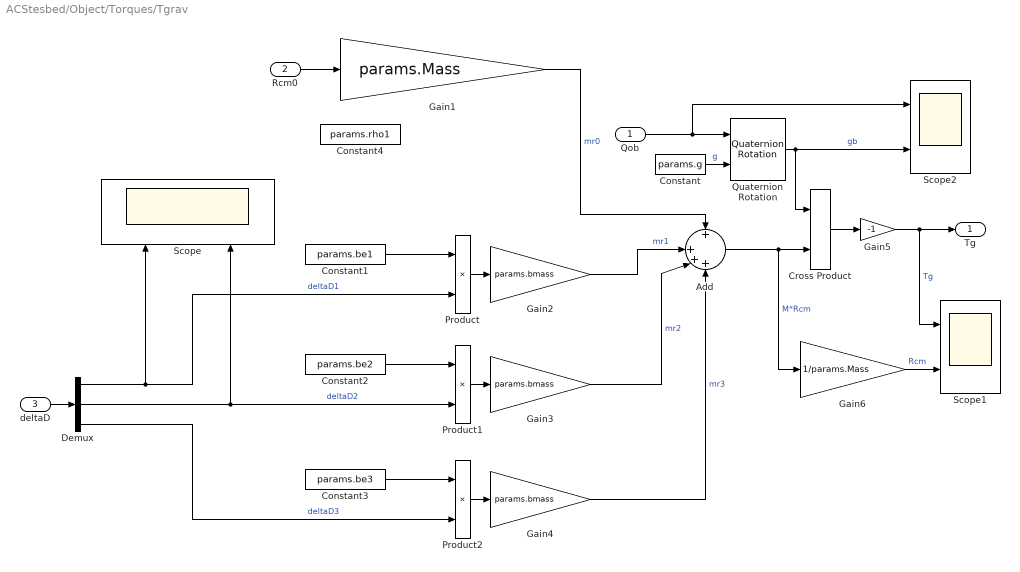
== system ACStesbed/Object/Torques/Tgrav ==
  Qob : Inport
  Rcm0 : Inport  Port=2
  deltaD : Inport  Port=3
  Add : Sum  Inputs=+|+++
  Constant : Constant  Value=params.g
  Constant1 : Constant  Value=params.be1
  Constant2 : Constant  Value=params.be2
  Constant3 : Constant  Value=params.be3
  Constant4 : Constant  Value=params.rho1
  Cross Product : vrlib/Utilities/Cross Product
  Demux : Demux  Outputs=3
  Gain1 : Gain  Gain=params.Mass
  Gain2 : Gain  Gain=params.bmass
  Gain3 : Gain  Gain=params.bmass
  Gain4 : Gain  Gain=params.bmass
  Gain5 : Gain  Gain=-1
  Gain6 : Gain  Gain=1/params.Mass
  Product : Product
  Product1 : Product
  Product2 : Product
  Quaternion Rotation : aerolibutil/Quaternion Rotation
  Scope : Scope  NumInputPorts=2
  Scope1 : Scope  NumInputPorts=2
  Scope2 : Scope  NumInputPorts=2
  Tg : Outport
  wires:
  Rcm0/1 -> Gain1/1
  Constant/1 -> Quaternion Rotation/2  "g"
  Gain1/1 -> Add/1  "mr0"
  Constant1/1 -> Product/1
  deltaD/1 -> Demux/1
  Constant2/1 -> Product1/1
  Demux/2 -> Scope/2, Product1/2  "deltaD2"
  Constant3/1 -> Product2/1
  Product/1 -> Gain2/1
  Product1/1 -> Gain3/1
  Product2/1 -> Gain4/1
  Gain2/1 -> Add/2  "mr1"
  Gain3/1 -> Add/3  "mr2"
  Gain4/1 -> Add/4  "mr3"
  Add/1 -> Cross Product/2, Gain6/1  "M*Rcm"
  Demux/3 -> Product2/2  "deltaD3"
  Demux/1 -> Scope/1, Product/2  "deltaD1"
  Quaternion Rotation/1 -> Cross Product/1, Scope2/2  "gb"
  Cross Product/1 -> Gain5/1
  Gain5/1 -> Scope1/1, Tg/1  "Tg"
  Qob/1 -> Scope2/1, Quaternion Rotation/1
  Gain6/1 -> Scope1/2  "Rcm"

== system ACStesbed/Object/Torques/Tm ==
  L : Inport
  B : Inport  Port=2
  Ldisturb : Inport  Port=3
  Tm : Outport
  wires:
  L/1 -> Tm/1

== system ACStesbed/Object/Torques/Tothers ==
  Something : Inport
  Tothers : Outport
  wires:
  Something/1 -> Tothers/1

== system ACStesbed/Object/Torques/Trw ==
  dh : Inport
  W : Inport  Port=2
  h : Inport  Port=3
  Add : Sum
  Cross Product : vrlib/Utilities/Cross Product
  Gain : Gain  Gain=-1
  Trw : Outport
  wires:
  W/1 -> Cross Product/1
  Gain/1 -> Trw/1  "Trw"
  Cross Product/1 -> Add/2  "Wxh"
  Add/1 -> Gain/1  "(dH+WxH)"
  dh/1 -> Add/1
  h/1 -> Cross Product/2

== system ACStesbed/Sensors/SunSensor/DigitalSunSensor ==
  Rsun_ss : Inport
  Complex to Magnitude-Angle : ComplexToMagnitudeAngle
  Demux : Demux  Outputs=2
  Mux : Mux  Inputs=2
  Real-Imag to Complex : RealImagToComplex
  Selector : Selector  InputPortWidth=3  IndexOptions=Index vector (dialog)  Indices=[1 2]  OutputSizes=1
  Sum : Sum  Inputs=|++
  Sum1 : Sum  Inputs=++|
  Zero-Order Hold : ZeroOrderHold  SampleTime=params.SS_sample_time
  noise : Constant  Value=[0 0]
  noise1 : Constant  Value=[0 0]
  Sun_mag_angle_mes : Outport
  wires:
  Mux/1 -> Sun_mag_angle_mes/1  "Rsun_mes_b"
  Selector/1 -> Demux/1
  Demux/1 -> Real-Imag to Complex/1
  Demux/2 -> Real-Imag to Complex/2
  noise/1 -> Sum/2
  Complex to Magnitude-Angle/1 -> Sum1/2  "magnitude"
  Complex to Magnitude-Angle/2 -> Sum/1  "angle"
  noise1/1 -> Sum1/1
  Real-Imag to Complex/1 -> Complex to Magnitude-Angle/1
  Sum1/1 -> Mux/1
  Sum/1 -> Mux/2
  Zero-Order Hold/1 -> Selector/1
  Rsun_ss/1 -> Zero-Order Hold/1

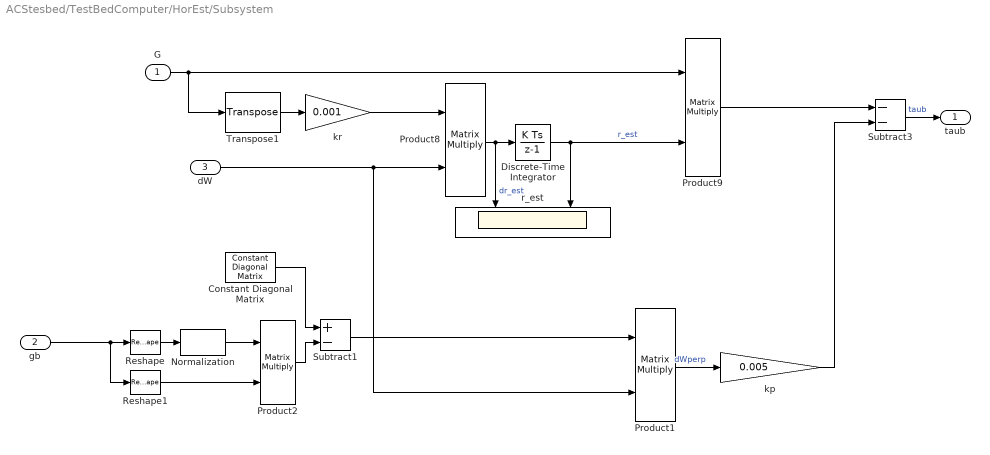
== system ACStesbed/TestBedComputer/HorEst/Subsystem ==
  G : Inport
  gb : Inport  Port=2
  dW : Inport  Port=3
  Constant Diagonal Matrix : dspmtrx3/Constant Diagonal Matrix  q=ones(1,3)  frame=off  dataType=Inherit from 'Constant(s) along diagonal'  isSigned=on  wordLen=16  udDataType=sfix(16)  fracBitsMode=Best precision  numFracBits=15
  Discrete-Time Integrator : DiscreteIntegrator  SampleTime=-1  ICPrevOutput=DiscIntNeverNeededParam  ICPrevScaledInput=DiscIntNeverNeededParam
  Normalization : dspmathops/Normalization  NormType=Squared 2-norm  Bias=1e-10  NormOver=Each column  ColComp=on  Dimension=1  outputDataTypeStr=Inherit: Same as product output  outputLastDataTypeStr=Inherit: Same as product output  outputMin=[]  outputMax=[]  accumDataTypeStr=Inherit: Same as product output  accumLastDataTypeStr=Inherit: Same as product output  roundingMode=Floor  overflowMode=off
  Product{1..2,8..9} (4 alike) : Product  Multiplication=Matrix(*)
  Reshape : Reshape  OutputDimensionality=Column vector (2-D)
  Reshape1 : Reshape  OutputDimensionality=Row vector (2-D)
  Subtract1 : Sum  Inputs=+-
  Subtract3 : Sum  Inputs=--
  Transpose1 : dspmtrx3/Transpose  Hermitian=off  overflowFlag=off
  kp : Gain  Gain=0.005
  kr : Gain  Gain=0.001
  r_est : Scope  NumInputPorts=2
  taub : Outport
  wires:
  Discrete-Time Integrator/1 -> Product9/2, r_est/2  "r_est"
  Product8/1 -> Discrete-Time Integrator/1, r_est/1  "dr_est"
  dW/1 -> Product1/2, Product8/2
  G/1 -> Product9/1, Transpose1/1
  Subtract3/1 -> taub/1  "taub"
  gb/1 -> Reshape1/1, Reshape/1
  Constant Diagonal Matrix/1 -> Subtract1/1
  Reshape1/1 -> Product2/2
  Reshape/1 -> Normalization/1
  Product2/1 -> Subtract1/2
  Normalization/1 -> Product2/1
  Subtract1/1 -> Product1/1
  Product1/1 -> kp/1  "dWperp"
  kp/1 -> Subtract3/2
  Product9/1 -> Subtract3/1
  Transpose1/1 -> kr/1
  kr/1 -> Product8/1

== system ACStesbed/CentralComputer/ModelOfObject/Inertia/deltaJ1 ==
  d : Inport
  e : Inport  Port=2
  rho : Inport  Port=3
  Add : Sum
  Constant : Constant  Value=params.bmass
  Gain : Gain  Gain=-1
  Product : Product  Inputs=3
  Product1 : Product
  Skew-symmetric matrix : satellite_control_lib/Skew-symmetric matrix
  deltaJ : Outport
  wires:
  Constant/1 -> Gain/1
  e/1 -> Product1/2
  rho/1 -> Add/2
  Product/1 -> deltaJ/1  "(-m)[R x][R x]"
  Gain/1 -> Product/1
  d/1 -> Product1/1
  Product1/1 -> Add/1
  Add/1 -> Skew-symmetric matrix/1  "R"
  Skew-symmetric matrix/1 -> Product/3, Product/2

== system ACStesbed/CentralComputer/ModelOfObject/Inertia/deltaJ2 ==
  d : Inport
  e : Inport  Port=2
  rho : Inport  Port=3
  Add : Sum
  Constant : Constant  Value=params.bmass
  Gain : Gain  Gain=-1
  Product : Product  Inputs=3
  Product1 : Product
  Skew-symmetric matrix : satellite_control_lib/Skew-symmetric matrix
  deltaJ : Outport
  wires:
  Skew-symmetric matrix/1 -> Product/2, Product/3
  Add/1 -> Skew-symmetric matrix/1  "R"
  Product1/1 -> Add/1
  d/1 -> Product1/1
  Gain/1 -> Product/1
  Product/1 -> deltaJ/1  "(-m)[R x][R x]"
  rho/1 -> Add/2
  e/1 -> Product1/2
  Constant/1 -> Gain/1

== system ACStesbed/CentralComputer/ModelOfObject/Inertia/deltaJ3 ==
  d : Inport
  e : Inport  Port=2
  rho : Inport  Port=3
  Add : Sum
  Constant : Constant  Value=params.bmass
  Gain : Gain  Gain=-1
  Product : Product  Inputs=3
  Product1 : Product
  Skew-symmetric matrix : satellite_control_lib/Skew-symmetric matrix
  deltaJ : Outport
  wires:
  Constant/1 -> Gain/1
  e/1 -> Product1/2
  rho/1 -> Add/2
  Product/1 -> deltaJ/1  "(-m)[R x][R x]"
  Gain/1 -> Product/1
  d/1 -> Product1/1
  Product1/1 -> Add/1
  Add/1 -> Skew-symmetric matrix/1  "R"
  Skew-symmetric matrix/1 -> Product/3, Product/2

== system ACStesbed/CentralComputer/SatAttitude/BINS/BINS correction ==
  Qjb_starmes : Inport
  Qjb_mes : Inport  Port=2
  Quaternion Conjugate : aerolibutil/Quaternion Conjugate
  Quaternion Conjugate1 : aerolibutil/Quaternion Conjugate
  Quaternion Multiplication : aerolibutil/Quaternion Multiplication
  Quaternion Multiplication1 : aerolibutil/Quaternion Multiplication
  Qjb_corrected : Outport
  wires:
  Quaternion Multiplication1/1 -> Qjb_corrected/1  "Qjb_corrected"
  Quaternion Conjugate1/1 -> Quaternion Multiplication1/1
  Qjb_mes/1 -> Quaternion Multiplication1/2, Quaternion Multiplication/2
  Quaternion Multiplication/1 -> Quaternion Conjugate1/1  "Nbb_mes"
  Qjb_starmes/1 -> Quaternion Conjugate/1
  Quaternion Conjugate/1 -> Quaternion Multiplication/1  "conjQjb_starmes"

== system ACStesbed/CentralComputer/SatAttitude/BINS/Calc Qob ==
  Qjo : Inport
  Qjb : Inport  Port=2
  Quaternion Inverse : aerolibutil/Quaternion Inverse
  Quaternion Multiplication : aerolibutil/Quaternion Multiplication
  Qob : Outport
  wires:
  Qjb/1 -> Quaternion Multiplication/2  "Qjb"
  Qjo/1 -> Quaternion Inverse/1  "Qjo"
  Quaternion Inverse/1 -> Quaternion Multiplication/1
  Quaternion Multiplication/1 -> Qob/1

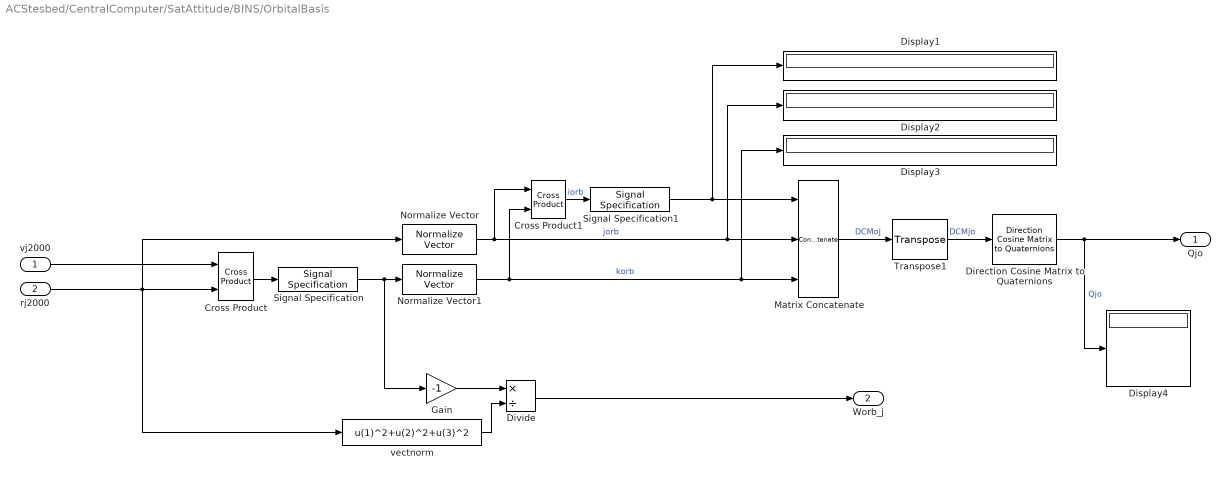
== system ACStesbed/CentralComputer/SatAttitude/BINS/OrbitalBasis ==
  vj2000 : Inport
  rj2000 : Inport  Port=2
  Cross Product : vrlib/Utilities/Cross Product
  Cross Product1 : vrlib/Utilities/Cross Product
  Direction Cosine Matrix to Quaternions : aerolibtransform2/Direction Cosine Matrix  to Quaternions
  Display{1..4} (4 alike) : Display
  Divide : Product  Inputs=*/
  Gain : Gain  Gain=-1
  Matrix Concatenate : Concatenate  NumInputs=3  Mode=Multidimensional array  ConcatenateDimension=2
  Normalize Vector : vrlib/Utilities/Normalize Vector  maxzero=0.00001
  Normalize Vector1 : vrlib/Utilities/Normalize Vector  maxzero=0.00001
  Signal Specification : SignalSpecification  Dimensions=3
  Signal Specification1 : SignalSpecification  Dimensions=3
  Transpose1 : dspmtrx3/Transpose  Hermitian=off  overflowFlag=off
  vectnorm : Fcn  Expr=u(1)^2+u(2)^2+u(3)^2
  Qjo : Outport
  Worb_j : Outport  Port=2
  wires:
  Cross Product1/1 -> Signal Specification1/1  "iorb"
  Normalize Vector/1 -> Display2/1, Matrix Concatenate/2, Cross Product1/1  "jorb"
  Matrix Concatenate/1 -> Transpose1/1  "DCMoj"
  rj2000/1 -> Cross Product/2, Normalize Vector/1, vectnorm/1
  vj2000/1 -> Cross Product/1
  Direction Cosine Matrix to Quaternions/1 -> Display4/1, Qjo/1  "Qjo"
  Normalize Vector1/1 -> Display3/1, Matrix Concatenate/3, Cross Product1/2  "korb"
  Cross Product/1 -> Signal Specification/1
  Gain/1 -> Divide/1
  vectnorm/1 -> Divide/2
  Divide/1 -> Worb_j/1
  Signal Specification/1 -> Gain/1, Normalize Vector1/1
  Signal Specification1/1 -> Display1/1, Matrix Concatenate/1
  Transpose1/1 -> Direction Cosine Matrix to Quaternions/1  "DCMjo"

== system ACStesbed/CentralComputer/SatAttitude/BINS/SIgnQuat ==
  Q : Inport
  Product : Product
  Selector2 : Selector  InputPortWidth=4  IndexOptions=Index vector (dialog)  Indices=[1]  OutputSizes=1
  Sign : Signum
  Q' : Outport
  wires:
  Q/1 -> Product/2, Selector2/1
  Product/1 -> Q'/1
  Sign/1 -> Product/1
  Selector2/1 -> Sign/1

== system ACStesbed/CentralComputer/SatAttitude/BINS/SIgnQuat1 ==
  Q : Inport
  Constant : Constant
  Constant1 : Constant  Value=-1
  Product : Product
  Selector2 : Selector  InputPortWidth=4  IndexOptions=Index vector (dialog)  Indices=[1]  OutputSizes=1
  Switch : Switch
  Q' : Outport
  wires:
  Q/1 -> Product/2, Selector2/1
  Product/1 -> Q'/1
  Switch/1 -> Product/1
  Selector2/1 -> Switch/2
  Constant/1 -> Switch/1
  Constant1/1 -> Switch/3

== system ACStesbed/CentralComputer/SatAttitude/BINS/SIgnQuat2 ==
  Q : Inport
  Constant : Constant
  Constant1 : Constant  Value=-1
  Product : Product
  Selector2 : Selector  InputPortWidth=4  IndexOptions=Index vector (dialog)  Indices=[1]  OutputSizes=1
  Switch : Switch
  Q' : Outport
  wires:
  Q/1 -> Product/2, Selector2/1
  Product/1 -> Q'/1
  Switch/1 -> Product/1
  Selector2/1 -> Switch/2
  Constant/1 -> Switch/1
  Constant1/1 -> Switch/3

== system ACStesbed/CentralComputer/SatAttitude/BINS/SIgnQuat3 ==
  Q : Inport
  Constant : Constant
  Constant1 : Constant  Value=-1
  Product : Product
  Selector2 : Selector  InputPortWidth=4  IndexOptions=Index vector (dialog)  Indices=[1]  OutputSizes=1
  Switch : Switch
  Q' : Outport
  wires:
  Q/1 -> Product/2, Selector2/1
  Product/1 -> Q'/1
  Switch/1 -> Product/1
  Selector2/1 -> Switch/2
  Constant/1 -> Switch/1
  Constant1/1 -> Switch/3

== system ACStesbed/CentralComputer/SatAttitude/BINS/SIgnQuat4 ==
  Q : Inport
  Constant : Constant
  Constant1 : Constant  Value=-1
  Product : Product
  Selector2 : Selector  InputPortWidth=4  IndexOptions=Index vector (dialog)  Indices=[1]  OutputSizes=1
  Switch : Switch
  Q' : Outport
  wires:
  Q/1 -> Product/2, Selector2/1
  Product/1 -> Q'/1
  Switch/1 -> Product/1
  Selector2/1 -> Switch/2
  Constant/1 -> Switch/1
  Constant1/1 -> Switch/3

== system ACStesbed/CentralComputer/SatAttitude/BINS/quatint ==
  p q r : Inport
  q_init : Inport  Port=2
  q0 q1 q2 q3 : Integrator  InitialConditionSource=external  InitialCondition=[e0_0 e1_0 e2_0 e3_0]
  qdot : aerolib6dofsys/DCM & Euler Angles (Quaternion)/qdot
  q : Outport
  wires:
  q0 q1 q2 q3/1 -> q/1, qdot/2
  q_init/1 -> q0 q1 q2 q3/2
  p q r/1 -> qdot/1
  qdot/1 -> q0 q1 q2 q3/1
